simulink model "AFKF_simulink"  (R2018a)
settings: Solver=ode4  StartTime=0.0  StopTime=Data(end,1)  FixedStep=0.01  RelTol=1e-3
libraries: fuzblock x1
settings Model: Creator=emran  LastModifiedBy=emran

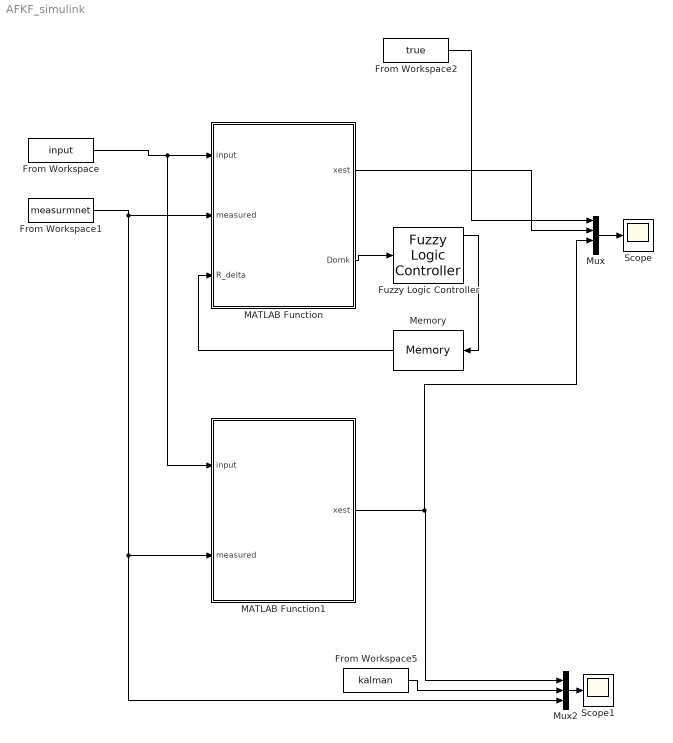
== system AFKF_simulink ==
  From Workspace : FromWorkspace  VariableName=input  SampleTime=0
  From Workspace1 : FromWorkspace  VariableName=measurmnet  SampleTime=0
  From Workspace2 : FromWorkspace  VariableName=true  SampleTime=0
  From Workspace5 : FromWorkspace  VariableName=kalman  SampleTime=0
  Fuzzy Logic Controller : fuzblock/Fuzzy Logic  Controller  FIS='FAKF.fis'  OutputSampleNumber=101  DataType=double  FuzzifiedInputs=on  RuleFiringStrengths=on  RuleOutputs=off  AggregatedOutputs=off  SimulateUsing=Interpreted execution  OutOfRangeInputValueMessage=warning  NoRuleFiredMessage=warning  EmptyOutputFuzzySetMessage=warning
  MATLAB Function : MATLAB Function  TreatAsAtomicUnit=on
  MATLAB Function1 : MATLAB Function  TreatAsAtomicUnit=on
  Memory : Memory
  Mux : Mux
  Mux2 : Mux  Inputs=3
  Scope : Scope
  Scope1 : Scope
  wires:
  MATLAB Function/2(Domk) -> Fuzzy Logic Controller/1
  Fuzzy Logic Controller/1 -> Memory/1
  Memory/1 -> MATLAB Function/3(R_delta)
  MATLAB Function/1(xest) -> Mux/2
  MATLAB Function1/1(xest) -> Mux/3, Mux2/1
  Mux/1 -> Scope/1
  Mux2/1 -> Scope1/1
  From Workspace5/1 -> Mux2/2
  From Workspace1/1 -> MATLAB Function/2(measured), Mux2/3, MATLAB Function1/2(measured)
  From Workspace2/1 -> Mux/1
  From Workspace/1 -> MATLAB Function1/1(input), MATLAB Function/1(input)

== matlab function AFKF_simulink/MATLAB Function1 ==
  settings: updateMethod=DISCRETE
  data: xest output; input input; measured input
function xest  = fcn(input, measured)
persistent xh P
if isempty(xh)
    xh = [0; 0];
    P = eye(2);
end

%% Kalman Declaration        
Ad = [0.9998 0.009851; -0.0394 0.9702];
Bd = [0.000198; 0.0394];
Cd = [1 0];

Q = 1;
R = diag([0.25,5]);
%% Kalman Procedure

% Model information
xh_bar = Ad * xh + Bd * input;
P_bar  = Ad * P * Ad' + R;

% Measurement update

K  = P_bar * Cd' * (Cd * P_bar * Cd' + Q)^-1;
xh = xh_bar +  K * (measured - Cd * xh_bar);
P  = (1 - K * Cd) * P_bar;
xest = Cd * xh;

== matlab function AFKF_simulink/MATLAB Function ==
  settings: updateMethod=DISCRETE
  data: xest output; Domk output; input input; measured input; R_delta input
function [xest, Domk] = fcn(input, measured, R_delta)
persistent xh P R Crk
if isempty(xh)
    xh = [0; 0];
    P = eye(2);
    R = diag([0.2,5]);
    Crk = 0;
end
R(1) = R(1) + 0.001 * R_delta;

%% Kalman Declaration
N = 50; % estimation window
        
Ad = [0.9998 0.009851; -0.0394 0.9702];
Bd = [0.000198; 0.0394];
Cd = [1 0];

Q = 1;
%% Kalman Procedure
Ts = 0.0001;
% Model information
xh_bar = xh + (Ad * xh + Bd * input)*Ts;
%xh_bar = Ad * xh + Bd * input;
P_bar  = Ad * P * Ad' + R;

% Measurement update

K  = P_bar * Cd' * (Cd * P_bar * Cd' + Q)^-1;
S  =                Cd * P_bar * Cd' + Q;
xh = xh_bar +  K * (measured - Cd * xh_bar);
P  = (1 - K * Cd) * P_bar;
xest = Cd * xh;
% R matrix adaptation
r = Cd * xh_bar;

% Fuzzy code begins 
%for s= counter-N+1:counter 
% Crk=Crk+((r)*(r)'/N);
%Crk=(r*r'/N);
%end

for s = 1:N 
Crk = Crk + ((r)*(r)'/N);
end

DoM = S(1,1) - Crk(1,1);% deg of Matching 
Domk= 2 * DoM; % Input for the FIS
Domk= min(max(Domk,-10),10);
